simulink model "mmcs_s2f"  (R2021b)
settings: Solver=FixedStepDiscrete  StartTime=0.0  StopTime=5  FixedStep=T_HF_TASK  RelTol=1e-3  EnableMultiTasking=on
PostLoadFcn:
  | run('init.m')
values from neighbouring files (symbols this model uses):
  ALIGN_DURATION = 700.0    [mmcs_s2f_dd.sldd]
  ALIGN_FINAL_CURRENT = 3277.0    [mmcs_s2f_dd.sldd]
  ALIGN_FINAL_SPEED = 0.0    [mmcs_s2f_dd.sldd]
  ALIGN_INIT_CURRENT = 1638.0    [mmcs_s2f_dd.sldd]
  ALIGN_THETA = 2731.0    [mmcs_s2f_dd.sldd]
  AMPTOS16 = 3277.0    [mmcs_s2f_dd.sldd]
  DIVSQRT_3 = 18918.0    [mmcs_s2f_dd.sldd]
  ENC_PT_CTRL = 4.0    [mmcs_s2f_dd.sldd]
  ENC_PULSE_NUM = 4000    [mmcs_s2f_dd.sldd]
  ENC_ST_CTRL = 2.0    [mmcs_s2f_dd.sldd]
  IF_ACC_DURATION = 1500.0    [mmcs_s2f_dd.sldd]
  IF_FINAL_CURRENT = 3277.0    [mmcs_s2f_dd.sldd]
  IF_FINAL_CURRENT_LOL = -3277.0    [mmcs_s2f_dd.sldd]
  IF_FINAL_CURRENT_UPL = 3277.0    [mmcs_s2f_dd.sldd]
  IF_FINAL_SPEED = 600.0    [mmcs_s2f_dd.sldd]
  IF_FINAL_SPEED_LOL = -600.0    [mmcs_s2f_dd.sldd]
  IF_FINAL_SPEED_UPL = 600.0    [mmcs_s2f_dd.sldd]
  IF_INIT_CURRENT = 1638.0    [mmcs_s2f_dd.sldd]
  INT16_MAX = 32767.0    [mmcs_s2f_dd.sldd]
  INT16_MIN = -32768.0    [mmcs_s2f_dd.sldd]
  MOTOR_F = 7.0E-6    [mmcs_s2f_dd.sldd]
  MOTOR_J = 2.8E-6    [mmcs_s2f_dd.sldd]
  MOTOR_PN = 4    [mmcs_s2f_dd.sldd]
  MOTOR_PNF = 4.0    [mmcs_s2f_dd.sldd]
  MOTOR_TL = 0.001    [mmcs_s2f_dd.sldd]
  PI_KI_PLL : value not decoded    [mmcs_s2f_dd.sldd]
  PI_KI_POS : value not decoded    [mmcs_s2f_dd.sldd]
  PI_KI_SPD : value not decoded    [mmcs_s2f_dd.sldd]
  PI_KI_TQ : value not decoded    [mmcs_s2f_dd.sldd]
  PI_KP_PLL : value not decoded    [mmcs_s2f_dd.sldd]
  PI_KP_POS : value not decoded    [mmcs_s2f_dd.sldd]
  PI_KP_SPD : value not decoded    [mmcs_s2f_dd.sldd]
  PI_KP_TQ : value not decoded    [mmcs_s2f_dd.sldd]
  PWM_FREQUENCY = 10000.0    [mmcs_s2f_dd.sldd]
  PWM_PERIOD_CYCLES = 7200.0    [mmcs_s2f_dd.sldd]
  RAD2RPM_F_DEN = 1000.0    [mmcs_s2f_dd.sldd]
  RAD2RPM_F_NUM = 9549.0    [mmcs_s2f_dd.sldd]
  RADTOS16_F = 10430.378350470453    [mmcs_s2f_dd.sldd]
  RADTOS16_I = 10430.0    [mmcs_s2f_dd.sldd]
  REF_CURRENT_LOL = -11470.0    [mmcs_s2f_dd.sldd]
  REF_CURRENT_UPL = 11470.0    [mmcs_s2f_dd.sldd]
  STM_ALIGN = 4.0    [mmcs_s2f_dd.sldd]
  STM_IFRUN = 5.0    [mmcs_s2f_dd.sldd]
  STM_INIT = 1.0    [mmcs_s2f_dd.sldd]
  STM_PTRUN = 7.0    [mmcs_s2f_dd.sldd]
  STM_START = 12.0    [mmcs_s2f_dd.sldd]
  STM_STRUN = 6.0    [mmcs_s2f_dd.sldd]
  STM_SWITCH = 11.0    [mmcs_s2f_dd.sldd]
  STO_C1 = 588    [mmcs_s2f_dd.sldd]
  STO_C2 = -5703    [mmcs_s2f_dd.sldd]
  STO_C3 = 1554    [mmcs_s2f_dd.sldd]
  STO_C4 = 7484    [mmcs_s2f_dd.sldd]
  STO_C5 = 1831    [mmcs_s2f_dd.sldd]
  STO_EST_MAX = 134213632.0    [mmcs_s2f_dd.sldd]
  STO_EST_MIN = -134213632.0    [mmcs_s2f_dd.sldd]
  STO_F1 = 4096.0    [mmcs_s2f_dd.sldd]
  STO_F2 = 4096.0    [mmcs_s2f_dd.sldd]
  STO_ST_CTRL = 3.0    [mmcs_s2f_dd.sldd]
  STOMS = 1000.0    [mmcs_s2f_dd.sldd]
  T_HF_TASK = 0.0001    [mmcs_s2f_dd.sldd]
  T_MF_TASK = 0.002    [mmcs_s2f_dd.sldd]
  TORQ_CTRL = 0.0    [mmcs_s2f_dd.sldd]
  U32MAXdivPulseNumber = 1073741    [mmcs_s2f_dd.sldd]
  VBUS = 24.0    [mmcs_s2f_dd.sldd]
undefined symbols (not defined in the file or in its folder): DiscIntNeverNeededParam
libraries: simulink x22, slpidlib x5, mcbplantlib x1, autolibpmsmexterior x1
(part 1 of 5)
settings Model: DataDictionary=mmcs_s2f_dd.sldd  FPTShortcutValueString='{{},{''BaselineRun_3'',1,1,1,''BaselineRun_3'','''',{},''M'','''',''''},{''BaselineRun_4'',1,1,1,''BaselineRun_4'','''',{},''M'','''',''''}}'  PacingRate=0.500000  Creator=lww186  LastModifiedBy=lww186
settings SolverCC: AutoInsertRateTranBlk=on
settings OptimizationCC: DefaultParameterBehavior=Inlined  OptimizeBlockIOStorage=off  BufferReuse=off  GlobalBufferReuse=off  ExpressionFolding=off  EnableMemcpy=off  PassReuseOutputArgsAs=Individual arguments  LocalBlockOutputs=off  ZeroExternalMemoryAtStartup=off  ZeroInternalMemoryAtStartup=off  OptimizeDataStoreBuffers=off  BusAssignmentInplaceUpdate=off  OptimizationLevel=level0  OptimizationPriority=Speed  OptimizationCustomize=off  EfficientTunableParamExpr=on
settings DebuggingCC: SignalRangeChecking=warning  InheritedTsInSrcMsg=none  MultiTaskDSMMsg=none  ParameterPrecisionLossMsg=none
settings HardwareCC: ProdBitPerPointer=32  ProdBitPerSizeT=32  ProdBitPerPtrDiffT=32  ProdLargestAtomicInteger=Long  ProdLargestAtomicFloat=Double  ProdWordSize=32  ProdHWDeviceType=ARM Compatible->ARM Cortex-M
settings SFSimCC: MATLABDynamicMemAlloc=off
settings RTWCC: Description=Embedded Coder  SystemTargetFile=ert.tlc  GenCodeOnly=on  TemplateMakefile=ert_default_tmf  GenerateReport=on  LaunchReport=on
settings CodeAppCC: ForceParamTrailComments=on  IgnoreCustomStorageClasses=off  OperatorAnnotations=on  SimulinkDataObjDesc=on  SFDataObjDesc=on  InsertBlockDesc=on
settings ERTTargetCC: TargetLangStandard=C99 (ISO)  CodeReplacementLibrary=ARM Cortex-M  InlinedParameterPlacement=NonHierarchical  ERTCustomFileTemplate=example_file_process.tlc

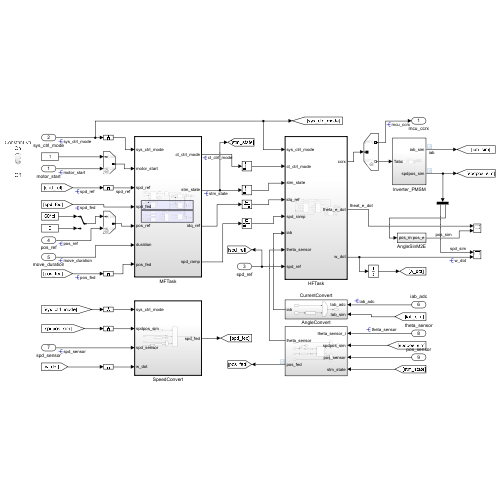
[thumbnail: Simulink's stored preview of the top-level diagram]
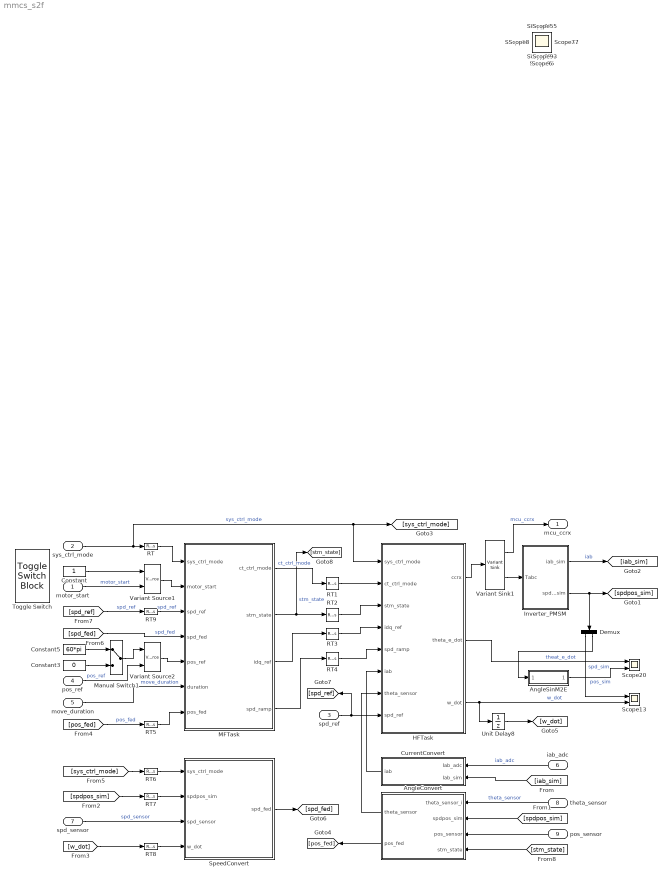
== system mmcs_s2f ==
  motor_start : Inport  OutDataTypeStr=uint8  LockScale=on
  sys_ctrl_mode : Inport  Port=2  OutDataTypeStr=uint8  LockScale=on
  spd_ref : Inport  Port=3  OutDataTypeStr=int16  LockScale=on
  pos_ref : Inport  Port=4  OutDataTypeStr=single  LockScale=on
  move_duration : Inport  Port=5  OutDataTypeStr=single  LockScale=on
  iab_adc : Inport  Port=6  OutDataTypeStr=int16  LockScale=on
  spd_sensor : Inport  Port=7  OutDataTypeStr=int16  LockScale=on
  theta_sensor : Inport  Port=8  OutDataTypeStr=int16
  pos_sensor : Inport  Port=9  OutDataTypeStr=int32
  AngleConvert : Subsystem  SystemSampleTime=T_HF_TASK
      settings: RTWFcnNameOpts=Use subsystem name  RTWFileNameOpts=Use subsystem name
  AngleSinM2E : Subsystem
  Constant : Constant  OutDataTypeStr=uint8
  Constant3 : Constant  Value=0  OutDataTypeStr=single
  Constant5 : Constant  Value=60*pi  OutDataTypeStr=single
  CurrentConvert : Subsystem  SystemSampleTime=T_HF_TASK
      settings: RTWFcnNameOpts=Use subsystem name  RTWFileNameOpts=Use subsystem name
  Demux : Demux  Outputs=2
  HFTask : Subsystem  TreatAsAtomicUnit=on  SystemSampleTime=T_HF_TASK
      settings: RTWFcnNameOpts=Use subsystem name  RTWFileNameOpts=Use subsystem name
  Inverter_PMSM : Subsystem
  MFTask : Subsystem  TreatAsAtomicUnit=on  SystemSampleTime=T_MF_TASK
      settings: RTWFcnNameOpts=Use subsystem name  RTWFileNameOpts=Use subsystem name
  Manual Switch1 : ManualSwitch
  RT{,5..9} (6 alike) : RateTransition  Deterministic=off  OutPortSampleTime=0.002
  RT{1..4} (4 alike) : RateTransition  Deterministic=off  OutPortSampleTime=0.0001
  Scope13 : Scope  NumInputPorts=2
  Scope20 : Scope  NumInputPorts=2
  SpeedConvert : Subsystem  TreatAsAtomicUnit=on  SystemSampleTime=T_MF_TASK
      settings: RTWFcnNameOpts=Use subsystem name  RTWFileNameOpts=Use subsystem name
  Toggle Switch : ToggleSwitchBlock
      settings: Values={{'Off', 'On'}, [0 1]}
  Unit Delay8 : UnitDelay  SampleTime=-1  HasFrameUpgradeWarning=on
  Variant Sink1 : VariantSink  VariantControlMode=sim codegen switching  ShowConditionOnBlock=on
  Variant Source1 : VariantSource  VariantControlMode=sim codegen switching  ShowConditionOnBlock=on
  Variant Source2 : VariantSource  VariantControlMode=sim codegen switching  ShowConditionOnBlock=on
  mcu_ccrx : Outport  OutDataTypeStr=uint16
  Scope{,1..12,14..19,21..37} (36 alike) : Scope
  wires:
  spd_ref/1 -> HFTask/8(spd_ref), [spd_ref]
  motor_start/1 -> Variant Source1/2  "motor_start"
  [iab_sim] -> CurrentConvert/2(Iab_sim)
  [spdpos_sim] -> AngleConvert/2(spdpos_sim)
  theta_sensor/1 -> AngleConvert/1(theta_sensor_i)  "theta_sensor"
  [spdpos_sim] -> RT7/1
  Inverter_PMSM/2(spdpos_sim) -> [spdpos_sim], Demux/1
  CurrentConvert/1(iab) -> HFTask/6(iab)
  Variant Sink1/1 -> mcu_ccrx/1  "mcu_ccrx"
  HFTask/1(ccrx) -> Variant Sink1/1
  Variant Sink1/2 -> Inverter_PMSM/1(Tabc)
  MFTask/3(idq_ref) -> RT3/1
  RT4/1 -> HFTask/5(spd_ramp)
  RT1/1 -> HFTask/2(ct_ctrl_mode)
  RT2/1 -> HFTask/3(stm_state)
  Variant Source1/1 -> MFTask/2(motor_start)
  pos_sensor/1 -> AngleConvert/3(pos_sensor)
  Constant/1 -> Variant Source1/1
  pos_ref/1 -> Variant Source2/2  "pos_ref"
  Variant Source2/1 -> MFTask/5(pos_ref)
  Manual Switch1/1 -> Variant Source2/1
  move_duration/1 -> MFTask/6(duration)  "move_duration"
  Constant5/1 -> Manual Switch1/1
  Constant3/1 -> Manual Switch1/2
  HFTask/3(w_dot) -> Unit Delay8/1, Scope13/2  "w_dot"
  [w_dot] -> RT8/1
  [sys_ctrl_mode] -> RT6/1
  HFTask/2(theta_e_dot) -> Scope20/1  "theat_e_dot"
  Unit Delay8/1 -> [w_dot]
  [spd_fed] -> MFTask/4(spd_fed)  "spd_fed"
  iab_adc/1 -> CurrentConvert/1(Iab_adc)  "iab_adc"
  AngleConvert/1(theta_sensor) -> HFTask/7(theta_sensor)
  Inverter_PMSM/1(iab_sim) -> [iab_sim]  "iab"
  SpeedConvert/1(spd_fed) -> [spd_fed]
  MFTask/1(ct_ctrl_mode) -> RT1/1  "ct_ctrl_mode"
  MFTask/2(stm_state) -> [stm_state], RT2/1  "stm_state"
  RT3/1 -> HFTask/4(idq_ref)
  MFTask/4(spd_ramp) -> RT4/1
  RT6/1 -> SpeedConvert/1(sys_ctrl_mode)
  RT7/1 -> SpeedConvert/2(spdpos_sim)
  RT8/1 -> SpeedConvert/4(w_dot)
  RT/1 -> MFTask/1(sys_ctrl_mode)
  RT5/1 -> MFTask/7(pos_fed)
  sys_ctrl_mode/1 -> HFTask/1(sys_ctrl_mode), [sys_ctrl_mode], RT/1  "sys_ctrl_mode"
  AngleSinM2E/1(pos_e) -> Scope20/2  "pos_sim"
  Demux/1 -> Scope13/1  "spd_sim"
  Demux/2 -> AngleSinM2E/1(pos_m)
  [spd_ref] -> RT9/1  "spd_ref"
  RT9/1 -> MFTask/3(spd_ref)  "spd_ref"
  spd_sensor/1 -> SpeedConvert/3(spd_sensor)  "spd_sensor"
  AngleConvert/2(pos_fed) -> [pos_fed]
  [pos_fed] -> RT5/1  "pos_fed"
  [stm_state] -> AngleConvert/4(stm_state)

== system mmcs_s2f/AngleConvert ==
  theta_sensor_i : Inport  OutDataTypeStr=int16
  spdpos_sim : Inport  Port=2  LockScale=on
  pos_sensor : Inport  Port=3  OutDataTypeStr=int32
  stm_state : Inport  Port=4  OutDataTypeStr=uint8
  Compare To Constant2 : simulink/Logic and Bit Operations/Compare To Constant  relop===  const=STM_ALIGN  OutDataTypeStr=uint8
  Demux : Demux  Outputs=2
      settings: DisplayOption=none
  EncCalcAngle : Subsystem
      settings: RTWFcnNameOpts=Use subsystem name  RTWFileNameOpts=Use subsystem name
  GetEncCnt : Subsystem  SystemSampleTime=T_HF_TASK
      settings: RTWFcnNameOpts=Use subsystem name  RTWFileNameOpts=Use subsystem name
  RT : RateTransition  Deterministic=off  OutPortSampleTime=0.0001
  Terminator : Terminator
  Variant Source : VariantSource  VariantControlMode=sim codegen switching  ShowConditionOnBlock=on
  Variant Source1 : VariantSource  VariantControlMode=sim codegen switching  ShowConditionOnBlock=on
  theta_sensor : Outport
  pos_fed : Outport  Port=2
  wires:
  spdpos_sim/1 -> Demux/1
  theta_sensor_i/1 -> Variant Source/1
  Variant Source/1 -> theta_sensor/1
  GetEncCnt/1(enc_cnt) -> EncCalcAngle/1(cnt)
  EncCalcAngle/1(theta_e_enc) -> Variant Source/2
  Demux/2 -> GetEncCnt/1(pos_sim)  "pos_sim"
  Demux/1 -> Terminator/1  "pos_sim"
  Variant Source1/1 -> pos_fed/1
  pos_sensor/1 -> Variant Source1/2
  EncCalcAngle/2(pos_fed) -> Variant Source1/1
  stm_state/1 -> Compare To Constant2/1
  Compare To Constant2/1 -> RT/1
  RT/1 -> EncCalcAngle/2(reset)

== system mmcs_s2f/AngleSinM2E ==
  pos_m : Inport
  AngleAbs2Sin : MATLAB Function  TreatAsAtomicUnit=on
  Constant2 : Constant  Value=MOTOR_PN
  Constant3 : Constant  Value=2*pi  OutDataTypeStr=single
  Data Type Conversion : DataTypeConversion  OutDataTypeStr=single  RndMeth=Zero
  Math Function1 : Math  Operator=rem  SaturateOnIntegerOverflow=on
  Product : Product  RndMeth=Zero
  pos_e : Outport  OutDataTypeStr=single
  wires:
  Math Function1/1 -> AngleAbs2Sin/1(u)
  Product/1 -> Math Function1/1
  Constant3/1 -> Math Function1/2
  Constant2/1 -> Product/2
  pos_m/1 -> Data Type Conversion/1
  Data Type Conversion/1 -> Product/1
  AngleAbs2Sin/1(y) -> pos_e/1

== system mmcs_s2f/CurrentConvert ==
  Iab_adc : Inport
  Iab_sim : Inport  Port=2
  Amp2s16A : Subsystem
  Variant Source1 : VariantSource  VariantControlMode=sim codegen switching  ShowConditionOnBlock=on
  iab : Outport
  wires:
  Iab_adc/1 -> Variant Source1/1
  Amp2s16A/1(Iab_s16A) -> Variant Source1/2
  Variant Source1/1 -> iab/1
  Iab_sim/1 -> Amp2s16A/1(Iab)

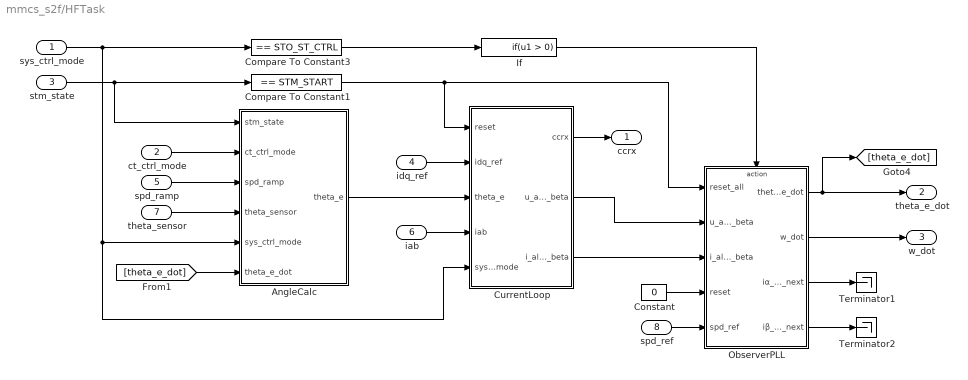
== system mmcs_s2f/HFTask ==
  sys_ctrl_mode : Inport  OutDataTypeStr=uint8
  ct_ctrl_mode : Inport  Port=2  OutDataTypeStr=uint8
  stm_state : Inport  Port=3  OutDataTypeStr=uint8
  idq_ref : Inport  Port=4  OutDataTypeStr=int16
  spd_ramp : Inport  Port=5  OutDataTypeStr=int16
  iab : Inport  Port=6  OutDataTypeStr=int16  LockScale=on
  theta_sensor : Inport  Port=7  OutDataTypeStr=int16  LockScale=on
  spd_ref : Inport  Port=8  OutDataTypeStr=int16
  AngleCalc : Subsystem  SystemSampleTime=T_HF_TASK
      settings: RTWFcnNameOpts=Use subsystem name  RTWFileNameOpts=Use subsystem name
  Compare To Constant1 : simulink/Logic and Bit Operations/Compare To Constant  relop===  const=STM_START  OutDataTypeStr=uint8
  Compare To Constant3 : simulink/Logic and Bit Operations/Compare To Constant  relop===  const=STO_ST_CTRL  OutDataTypeStr=uint8
  Constant : Constant  Value=0  OutDataTypeStr=uint8
  CurrentLoop : Subsystem  RTWFcnName=CurrentLoop  RTWFileName=CurrentLoop
      settings: RTWFcnNameOpts=Use subsystem name  RTWFileNameOpts=Use subsystem name
  If : If  ShowElse=off
  ObserverPLL : Subsystem  TreatAsAtomicUnit=on
      settings: RTWFcnNameOpts=Use subsystem name  RTWFileNameOpts=Use subsystem name
  Terminator1 : Terminator
  Terminator2 : Terminator
  ccrx : Outport  OutDataTypeStr=uint16
  theta_e_dot : Outport  Port=2  OutDataTypeStr=int16
  w_dot : Outport  Port=3  OutDataTypeStr=int16
  wires:
  idq_ref/1 -> CurrentLoop/2(idq_ref)
  AngleCalc/1(theta_e) -> CurrentLoop/3(theta_e)
  CurrentLoop/1(ccrx) -> ccrx/1
  spd_ramp/1 -> AngleCalc/3(spd_ramp)
  theta_sensor/1 -> AngleCalc/4(theta_sensor)
  ct_ctrl_mode/1 -> AngleCalc/2(ct_ctrl_mode)
  sys_ctrl_mode/1 -> Compare To Constant3/1, AngleCalc/5(sys_ctrl_mode), CurrentLoop/5(sys_ctrl_mode)
  Compare To Constant1/1 -> ObserverPLL/1(reset_all), CurrentLoop/1(reset)
  CurrentLoop/2(u_alhpa_beta) -> ObserverPLL/2(u_alpha_beta)
  CurrentLoop/3(i_alhpa_beta) -> ObserverPLL/3(i_alpha_beta)
  ObserverPLL/2(w_dot) -> w_dot/1
  [theta_e_dot] -> AngleCalc/6(theta_e_dot)
  ObserverPLL/1(theta_e_dot) -> [theta_e_dot], theta_e_dot/1
  iab/1 -> CurrentLoop/4(iab)
  stm_state/1 -> AngleCalc/1(stm_state), Compare To Constant1/1
  spd_ref/1 -> ObserverPLL/5(spd_ref)
  ObserverPLL/3(iα_dot_next) -> Terminator1/1
  ObserverPLL/4(iβ_dot_next) -> Terminator2/1
  Constant/1 -> ObserverPLL/4(reset)
  Compare To Constant3/1 -> If/1
  If/1 -> ObserverPLL/Action

== system mmcs_s2f/Inverter_PMSM ==
  Tabc : Inport
  Average-Value Inverter : mcbplantlib/Average-Value Inverter
  Bus Selector : BusSelector  OutputSignals=IaStator,IbStator,MtrSpd,MtrPos
  Constant1 : Constant  Value=MOTOR_TL  OutDataTypeStr=single
  Constant3 : Constant  Value=VBUS  OutDataTypeStr=single
  Mux1 : Mux  Inputs=2
  Mux2 : Mux  Inputs=2
  Surface Mount PMSM : autolibpmsmexterior/Surface Mount PMSM  port_config=Torque  sim_type=Discrete  Ts=T_HF_TASK  P=MOTOR_PNF  Rs=MOTOR_RS  Ldq_=MOTOR_LS  KConstText=Back-emf constant (Ke):  lambda_pm=0.2205  Ke=MOTOR_KE  Kt=1.323  mechanical=[MOTOR_J, MOTOR_F, 0]  idq0=[0 0]  theta_init=0  omega_init=0  KConst=0.2205  lambda_pm_calc=0.0077958  RefBlkName='autolibpmsmexterior/Surface Mount PMSM'  aMode=5  Ldq="[0.0017      0.0017]"
      settings: SourceProductBaseCode=PW,DR,MT,UV,VE
  Tabc2Dabc : Subsystem
  Terminator : Terminator
  Terminator1 : Terminator
  iab_sim : Outport
  spdpos_sim : Outport  Port=2
  wires:
  Tabc/1 -> Tabc2Dabc/1(Tabc)
  Tabc2Dabc/1(Dabc) -> Average-Value Inverter/1
  Constant3/1 -> Average-Value Inverter/2
  Average-Value Inverter/1 -> Surface Mount PMSM/2  "Vabc"
  Bus Selector/4 -> Mux1/2  "<MtrPos>"
  Constant1/1 -> Surface Mount PMSM/1  "load"
  Bus Selector/3 -> Mux1/1  "<MtrSpd>"
  Bus Selector/2 -> Mux2/2  "<IbStator>"
  Surface Mount PMSM/1 -> Bus Selector/1
  Mux2/1 -> iab_sim/1
  Bus Selector/1 -> Mux2/1  "<IaStator>"
  Mux1/1 -> spdpos_sim/1
  Surface Mount PMSM/2 -> Terminator/1
  Surface Mount PMSM/3 -> Terminator1/1

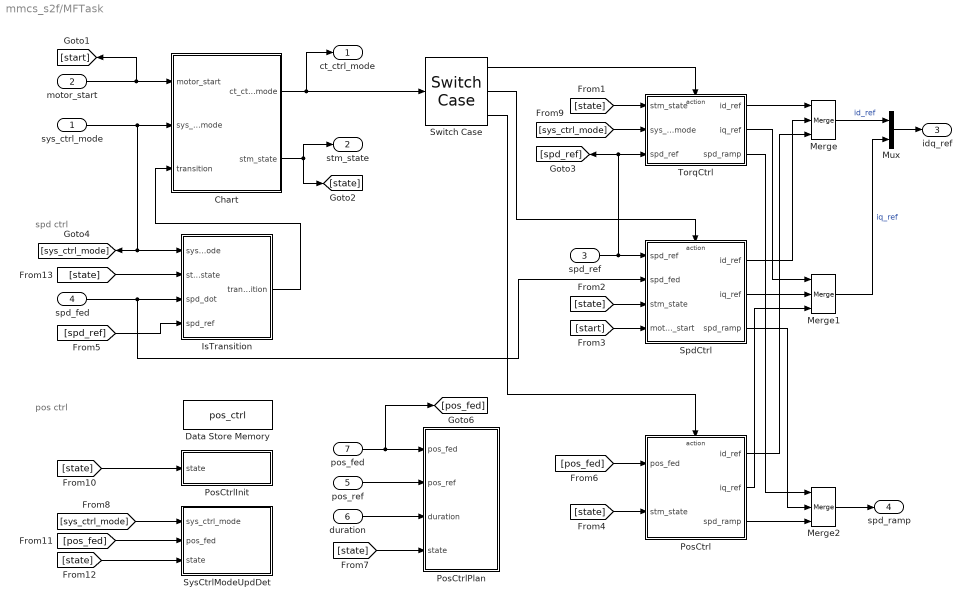
== system mmcs_s2f/MFTask ==
  note: pos ctrl
  note: spd ctrl
  sys_ctrl_mode : Inport  OutDataTypeStr=uint8
  motor_start : Inport  Port=2  OutDataTypeStr=uint8
  spd_ref : Inport  Port=3  OutDataTypeStr=int16
  spd_fed : Inport  Port=4  OutDataTypeStr=int16
  pos_ref : Inport  Port=5  OutDataTypeStr=single  LockScale=on
  duration : Inport  Port=6  OutDataTypeStr=single  LockScale=on
  pos_fed : Inport  Port=7  OutDataTypeStr=int32
  Chart : Stateflow chart
      settings: PortSchema="{\"entries\":[{\"content\":{\"sides\":[{\"content\":{\"connectorIds\":[\"In1\",\"In2\",\"In3\"]},\"type\":\"ConnectorPlacement.EquallySpacedRectSide\",\"uuid\":\"1a537016-921f-4174-a05c-35ab8fabf70c\"},{\"content\":{\"connectorIds\":[\"Out2\",\"Out1\"],\"side\":\"RIGHT\"},\"type\":\"ConnectorPlacement.EquallySpacedRectSide\",\"uuid\":\"0fdcb44e-8d7f-41bb-acf7-9927cd1be891\"},{\"content\":{\"connectorIds\":[],\"side\":\"TOP\"},\"type\":\"ConnectorPlacement.EquallySpacedRectSide\",\"uuid\":\"d2a61acf-9d71-44fa-a65c-bb3664d5d34b\"}]},\"type\":\"ConnectorPlacement.EquallySpacedConnector\",\"uuid\":\"a61f4b42-7cd9-4b03-82d8-8798bfa37e90\"}],\"packageUris\":[\"http://schema.mathworks.com/mf0/Connector/R2020b\"],\"version\":\"1.0\"}"
  Data Store Memory : DataStoreMemory  DataStoreName=pos_ctrl  ReadBeforeWriteMsg=warning  WriteAfterWriteMsg=warning  WriteAfterReadMsg=warning  ShowAdditionalParam=off  OutDataTypeStr=Bus: PosCtrlHandle_t
  IsTransition : Subsystem
      settings: RTWFcnNameOpts=Use subsystem name  RTWFileNameOpts=Use subsystem name
  Merge : Merge  Inputs=3
  Merge1 : Merge  Inputs=3
  Merge2 : Merge  Inputs=3
  Mux : Mux  Inputs=2
  PosCtrl : Subsystem  TreatAsAtomicUnit=on
  PosCtrlInit : Subsystem
  PosCtrlPlan : Subsystem
  SpdCtrl : Subsystem  TreatAsAtomicUnit=on
  Switch Case : SwitchCase  CaseConditions={TORQ_CTRL,SPD_CTRL,POS_CTRL}  ShowDefaultCase=off
  SysCtrlModeUpdDet : Subsystem
  TorqCtrl : Subsystem  TreatAsAtomicUnit=on
  ct_ctrl_mode : Outport  OutDataTypeStr=uint8
  stm_state : Outport  Port=2  OutDataTypeStr=uint8
  idq_ref : Outport  Port=3  OutDataTypeStr=int16
  spd_ramp : Outport  Port=4  OutDataTypeStr=int16
  wires:
  motor_start/1 -> Chart/1(motor_start), [start]
  Merge2/1 -> spd_ramp/1
  Switch Case/2 -> SpdCtrl/Action
  Chart/1(stm_state) -> [state], stm_state/1
  Merge1/1 -> Mux/2  "iq_ref"
  Merge/1 -> Mux/1  "id_ref"
  Chart/2(ct_ctrl_mode) -> ct_ctrl_mode/1, Switch Case/1
  Switch Case/1 -> TorqCtrl/Action
  [state] -> TorqCtrl/1(stm_state)
  spd_ref/1 -> SpdCtrl/1(spd_ref), TorqCtrl/3(spd_ref), [spd_ref]
  [state] -> SpdCtrl/3(stm_state)
  [start] -> SpdCtrl/4(motor_start)
  Switch Case/3 -> PosCtrl/Action
  spd_fed/1 -> SpdCtrl/2(spd_fed), IsTransition/3(spd_dot)
  TorqCtrl/1(id_ref) -> Merge/1
  SpdCtrl/1(id_ref) -> Merge/2
  PosCtrl/1(id_ref) -> Merge/3
  TorqCtrl/2(iq_ref) -> Merge1/1
  SpdCtrl/2(iq_ref) -> Merge1/2
  PosCtrl/2(iq_ref) -> Merge1/3
  TorqCtrl/3(spd_ramp) -> Merge2/1
  SpdCtrl/3(spd_ramp) -> Merge2/2
  PosCtrl/3(spd_ramp) -> Merge2/3
  [state] -> PosCtrl/2(stm_state)
  [sys_ctrl_mode] -> TorqCtrl/2(sys_ctrl_mode)
  [state] -> PosCtrlInit/1(state)
  pos_fed/1 -> [pos_fed], PosCtrlPlan/1(pos_fed)
  [pos_fed] -> PosCtrl/1(pos_fed)
  pos_ref/1 -> PosCtrlPlan/2(pos_ref)
  duration/1 -> PosCtrlPlan/3(duration)
  [state] -> PosCtrlPlan/4(state)
  [sys_ctrl_mode] -> SysCtrlModeUpdDet/1(sys_ctrl_mode)
  [pos_fed] -> SysCtrlModeUpdDet/2(pos_fed)
  [state] -> IsTransition/2(stm_state)
  IsTransition/1(transition) -> Chart/3(transition)
  sys_ctrl_mode/1 -> Chart/2(sys_ctrl_mode), [sys_ctrl_mode], IsTransition/1(sys_ctrl_mode)
  Mux/1 -> idq_ref/1
  [spd_ref] -> IsTransition/4(spd_ref)
  [state] -> SysCtrlModeUpdDet/3(state)

== system mmcs_s2f/SpeedConvert ==
  sys_ctrl_mode : Inport  OutDataTypeStr=uint8
  spdpos_sim : Inport  Port=2  OutDataTypeStr=double  LockScale=on
  spd_sensor : Inport  Port=3  OutDataTypeStr=int16  LockScale=on
  w_dot : Inport  Port=4  OutDataTypeStr=int16
  Constant2 : Constant  Value=STO_ST_CTRL  OutDataTypeStr=uint8
  Demux : Demux  Outputs=2
      settings: DisplayOption=none
  Relational Operator2 : RelationalOperator  Operator===  OutDataTypeStr=boolean  RndMeth=Zero
  SpdConvSim : Subsystem
  SpdConvSto : Subsystem
  Switch : Switch  Criteria=u2 > Threshold  RndMeth=Zero
  Terminator1 : Terminator
  Variant Source1 : VariantSource  VariantControlMode=sim codegen switching  ShowConditionOnBlock=on
  spd_fed : Outport  OutDataTypeStr=int16
  wires:
  spd_sensor/1 -> Variant Source1/1
  spdpos_sim/1 -> Demux/1
  sys_ctrl_mode/1 -> Relational Operator2/1
  w_dot/1 -> SpdConvSto/1(w_dot)
  Constant2/1 -> Relational Operator2/2
  SpdConvSto/1(spd_fed) -> Switch/1
  Demux/2 -> Terminator1/1
  Demux/1 -> SpdConvSim/1(spd_sim)
  Relational Operator2/1 -> Switch/2
  SpdConvSim/1(spd_fed) -> Variant Source1/2
  Variant Source1/1 -> Switch/3
  Switch/1 -> spd_fed/1

== system mmcs_s2f/AngleConvert/EncCalcAngle ==
  note: 1, theta_e
      |   - theta_e = cnt * U32MAXdivPulseNumber * Pn / 65536
      |   - U32MAXdivPulseNumber = 65536*65536/(1250*Pn)
      |   - theta_e Value rangef: [0~32767(pi), -32768(-pi)~0]
      | 2, pos_fed
      |   - theta_m = cnt * U32MAXdivPulseNumber / 65536
      |   - delta_theta_m = theta_m - theta_m_pre
      |   - pos_fed = The cumulative sum of delta_theta_m
      |   - uint: s16degree
  cnt : Inport  OutDataTypeStr=int32
  reset : Inport  Port=2  OutDataTypeStr=uint8
  Constant : Constant  Value=65536  OutDataTypeStr=int32
  Constant6 : Constant  Value=U32MAXdivPulseNumber  OutDataTypeStr=int32
  Data Type Conversion : DataTypeConversion  OutDataTypeStr=int16
  Data Type Conversion1 : DataTypeConversion  OutDataTypeStr=int16
  Discrete-Time Integrator : DiscreteIntegrator  IntegratorMethod=Accumulation: Forward Euler  ExternalReset=level  SampleTime=-1  OutDataTypeStr=int32  ICPrevOutput=DiscIntNeverNeededParam  ICPrevScaledInput=DiscIntNeverNeededParam
  Divide : Product  Inputs=*/  OutDataTypeStr=int32
  Gain5 : Gain  Gain=MOTOR_PN  OutDataTypeStr=int32
  Product2 : Product  OutDataTypeStr=int64
  Scope : Scope  NumInputPorts=4
  Subtract1 : Sum  Inputs=+-  AccumDataTypeStr=int16
  Unit Delay : UnitDelay  SampleTime=-1  HasFrameUpgradeWarning=on
  theta_e_enc : Outport  OutDataTypeStr=int16
  pos_fed : Outport  Port=2  OutDataTypeStr=int32
  wires:
  Constant6/1 -> Product2/2
  Product2/1 -> Scope/2, Divide/1
  cnt/1 -> Product2/1, Scope/1
  Constant/1 -> Divide/2
  Gain5/1 -> Data Type Conversion/1
  Unit Delay/1 -> Subtract1/2  "theta_m_pre"
  Data Type Conversion1/1 -> Subtract1/1, Unit Delay/1, Gain5/1, Scope/3  "theta_m"
  Discrete-Time Integrator/1 -> pos_fed/1
  Subtract1/1 -> Discrete-Time Integrator/1  "delta_theta_m"
  reset/1 -> Discrete-Time Integrator/2
  Data Type Conversion/1 -> Scope/4, theta_e_enc/1  "theta_e"
  Divide/1 -> Data Type Conversion1/1

== system mmcs_s2f/AngleConvert/GetEncCnt ==
  pos_sim : Inport  LockScale=on
  Add1 : Sum  RndMeth=Zero
  Constant1 : Constant  Value=2*pi
  Divide : Product  Inputs=*/  OutDataTypeStr=int32  RndMeth=Zero
  Gain3 : Gain  Gain=ENC_PULSE_NUM  RndMeth=Zero
  Math Function : Math  Operator=mod  SaturateOnIntegerOverflow=on
  Scope : Scope  NumInputPorts=2
  enc_cnt : Outport
  wires:
  Divide/1 -> enc_cnt/1, Scope/2
  Constant1/1 -> Math Function/2, Divide/2, Add1/2
  Gain3/1 -> Divide/1
  Add1/1 -> Math Function/1
  Math Function/1 -> Gain3/1
  pos_sim/1 -> Add1/1, Scope/1  "pos_sim"

== system mmcs_s2f/CurrentConvert/Amp2s16A ==
  Iab : Inport
  Data Type Conversion : DataTypeConversion  OutDataTypeStr=int16  RndMeth=Zero
  Gain : Gain  Gain=AMPTOS16  OutDataTypeStr=int32  RndMeth=Zero
  Saturation : Saturate  UpperLimit=INT16_MAX  LowerLimit=INT16_MIN  RndMeth=Zero
  Iab_s16A : Outport  OutDataTypeStr=int16
  wires:
  Iab/1 -> Gain/1
  Gain/1 -> Saturation/1
  Saturation/1 -> Data Type Conversion/1
  Data Type Conversion/1 -> Iab_s16A/1

== system mmcs_s2f/HFTask/AngleCalc ==
  stm_state : Inport  OutDataTypeStr=uint8
  ct_ctrl_mode : Inport  Port=2  OutDataTypeStr=uint8
  spd_ramp : Inport  Port=3  OutDataTypeStr=int16
  theta_sensor : Inport  Port=4  OutDataTypeStr=int16
  sys_ctrl_mode : Inport  Port=5  OutDataTypeStr=uint8
  theta_e_dot : Inport  Port=6  OutDataTypeStr=int16
  Constant1 : Constant  Value=TORQ_CTRL  OutDataTypeStr=uint8
  Constant2 : Constant  Value=STO_ST_CTRL  OutDataTypeStr=uint8
  Relational Operator1 : RelationalOperator  Operator===  OutDataTypeStr=boolean  RndMeth=Zero
  Relational Operator2 : RelationalOperator  Operator===  OutDataTypeStr=boolean  RndMeth=Zero
  Switch : Switch  Criteria=u2 > Threshold  RndMeth=Zero
  Switch1 : Switch  Criteria=u2 > Threshold  RndMeth=Zero
  VssCalcAngle : Subsystem
      settings: RTWFcnNameOpts=Use subsystem name  RTWFileNameOpts=Use subsystem name
  theta_e : Outport
  wires:
  spd_ramp/1 -> VssCalcAngle/2(spd_ramp)
  theta_sensor/1 -> Switch/3
  Constant2/1 -> Relational Operator2/2
  Relational Operator2/1 -> Switch/2
  sys_ctrl_mode/1 -> VssCalcAngle/3(sys_ctrl_mode), Relational Operator2/1
  theta_e_dot/1 -> Switch/1
  Switch/1 -> Switch1/3
  VssCalcAngle/1(theta_e) -> Switch1/1
  ct_ctrl_mode/1 -> Relational Operator1/1
  Relational Operator1/1 -> Switch1/2
  Constant1/1 -> Relational Operator1/2
  Switch1/1 -> theta_e/1
  stm_state/1 -> VssCalcAngle/1(stm_state)
